simulink model "qpsk"  (R2018a)
settings: Solver=VariableStepAuto  StartTime=0.0  StopTime=10.0  RelTol=1e-3
libraries: commdigbbndpm3 x2, commchan3 x1, commsink2 x1, commrandsrc3 x1
settings Model: Creator=user  LastModifiedBy=user

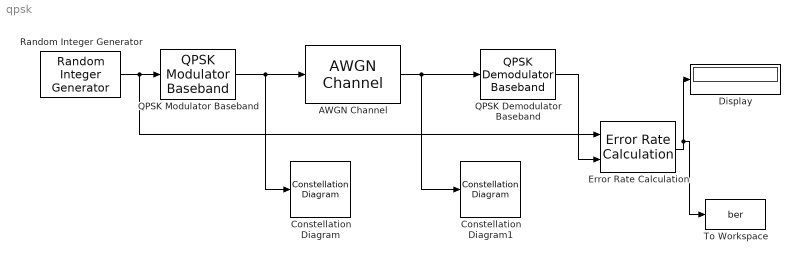
== system qpsk ==
  AWGN Channel : commchan3/AWGN Channel  InputProcessing=Columns as channels (frame based)  seed=67  noiseMode="Signal to noise ratio  (Eb/No)"  EbNodB=EbNo  EsNodB=10  SNRdB=10  bitsPerSym=1  Ps=1  Tsym=1  variance=1
  Constellation Diagram : ConstellationDiagram
  Constellation Diagram1 : ConstellationDiagram
  Display : Display
  Error Rate Calculation : commsink2/Error Rate Calculation  N=0  st_delay=0  cp_mode=Entire frame  subframe=[]  PMode=Port  WsName=ErrorVec  RsMode2=off  stop=off  numErr=100  maxBits=1e6
  QPSK Demodulator Baseband : commdigbbndpm3/QPSK Demodulator Baseband  OutType=Integer  DecType=Hard decision  VarSource=Dialog  Variance=1  Dec=Gray  Ph=pi/4  outDtype1=Inherit via internal rule  outDtype2=Inherit via internal rule  derotateFactorWordLen=16  derotateFactorDataTypeStr=Inherit: Same word length as input  derotateFactorLastDataTypeStr=Inherit: Same word length as input
  QPSK Modulator Baseband : commdigbbndpm3/QPSK Modulator Baseband  InType=Integer  Enc=Gray  Ph=pi/4  outDtype=double  outWordLen=16  outUDDataType=sfix(16)  outFracLenMode=Best precision  outFracLen=15  outDataTypeStr=double  outLastDataTypeStr=double
  Random Integer Generator : commrandsrc3/Random Integer Generator  SetSize=4  SeedSource=Parameter  Seed=37  SampleTime=1  SamplesPerFrame=100  OutputDataType=double  SimulateUsing=Interpreted execution
  To Workspace : ToWorkspace  VariableName=ber  SampleTime=-1
      settings: MaxDataPoints=2  Save2DSignal=2-D array (concatenate along first dimension)
  wires:
  Random Integer Generator/1 -> QPSK Modulator Baseband/1, Error Rate Calculation/1
  QPSK Modulator Baseband/1 -> Constellation Diagram/1, AWGN Channel/1
  AWGN Channel/1 -> QPSK Demodulator Baseband/1, Constellation Diagram1/1
  QPSK Demodulator Baseband/1 -> Error Rate Calculation/2
  Error Rate Calculation/1 -> To Workspace/1, Display/1
